simulink model "Kubon_lab8_1_sim"  (R2020b)
settings: Solver=VariableStepAuto  StartTime=0.0  StopTime=100.0  RelTol=1e-3
values from neighbouring files (symbols this model uses):
  A = [ (-cpN*ppN*fk0-ks1-k0)/(Cv1) , k0/Cv1 ; (k0+cpN*ppN*fk0)/(Cv2) , (-k0-cpN*ppN*fk0-ks2)/(Cv2)  ]    [Kubon_lab10.m]    (also in Kubon_lab8.m = [-a1/A1 , a1/A1 ; a1/A2 , (-a1-a2)/A2])
  B = [(cpN*ppN*fk0)/(Cv1) , ks2/Cv1 ; 0 , ks2/Cv2 ]    [Kubon_lab10.m]    (also in Kubon_lab8.m = [1/A1 , 0 ; 0 , 1/A2])
  C = eye(2)    [Kubon_lab10.m]    (also in Kubon_lab8.m)
  D = zeros(2)    [Kubon_lab10.m]    (also in Kubon_lab8.m)
  d1 = 0.1*fwe1max    [Kubon_lab6.m]    (also in Kubon_lab7.m = 0; Kubon_lab8.m = 0)
  d2 = 0.1*fwe2max    [Kubon_lab6.m]    (also in Kubon_lab7.m; Kubon_lab8.m)
  fwe1 = fwe1w(i)    [Kubon_lab6.m]    (also in Kubon_lab6_test.m; Kubon_lab7.m = 0.1*fwe1max; Kubon_lab8.m = 0.1*fwe1max)
  fwe2 = fwe2w(i)    [Kubon_lab6.m]    (also in Kubon_lab6_test.m; Kubon_lab7.m; Kubon_lab8.m)
  t0 = 50.0    (= 50)    [Kubon_lab10.m]    (also in Kubon_lab4.m = 5; Kubon_lab5.m = 0; Kubon_lab6.m = 5; Kubon_lab6_test.m = 0)
  x0 = 0    [Kubon_lab4.m]    (also in Kubon_lab5.m; Kubon_lab8.m = [h10,h20])
settings Model: Creator=pkubo  LastModifiedBy=pkubo

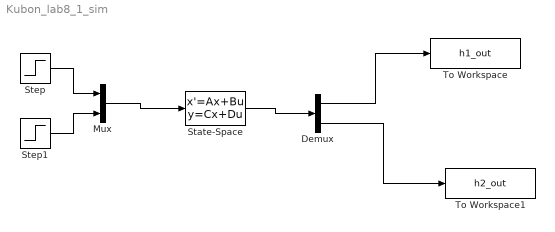
== system Kubon_lab8_1_sim ==
  Demux : Demux  Outputs=2
  Mux : Mux  Inputs=2
  State-Space : StateSpace  A=A  B=B  C=C  D=D  InitialCondition=x0
  Step : Step  Time=t0  Before=fwe1  After=fwe1+d1  SampleTime=0
  Step1 : Step  Time=t0  Before=fwe2  After=fwe2+d2  SampleTime=0
  To Workspace : ToWorkspace  VariableName=h1_out  SampleTime=-1
  To Workspace1 : ToWorkspace  VariableName=h2_out  SampleTime=-1
  wires:
  Step/1 -> Mux/1
  Step1/1 -> Mux/2
  Mux/1 -> State-Space/1
  State-Space/1 -> Demux/1
  Demux/1 -> To Workspace/1
  Demux/2 -> To Workspace1/1
